simulink model "Lazurit_VD_3x_V1"  (R2018b)
settings: Solver=ode8  StartTime=0.0  StopTime=0.2  RelTol=1e-3
undefined symbols (not defined in the file): C_c, C_r, L_l, L_r, R, Us, Uzpt
libraries: powerlib x36, powerlib_meascontrol x10, peRmsMeasurement x4
settings Model: Creator=Anton  LastModifiedBy=VID Company
settings SFSimCC: SimUseLocalCustomCode=off
settings RTWCC: RTWUseLocalCustomCode=off
settings CodeAppCC: StateflowObjectComments=on
settings SimscapeCC: SimscapeNormalizeSystem=off

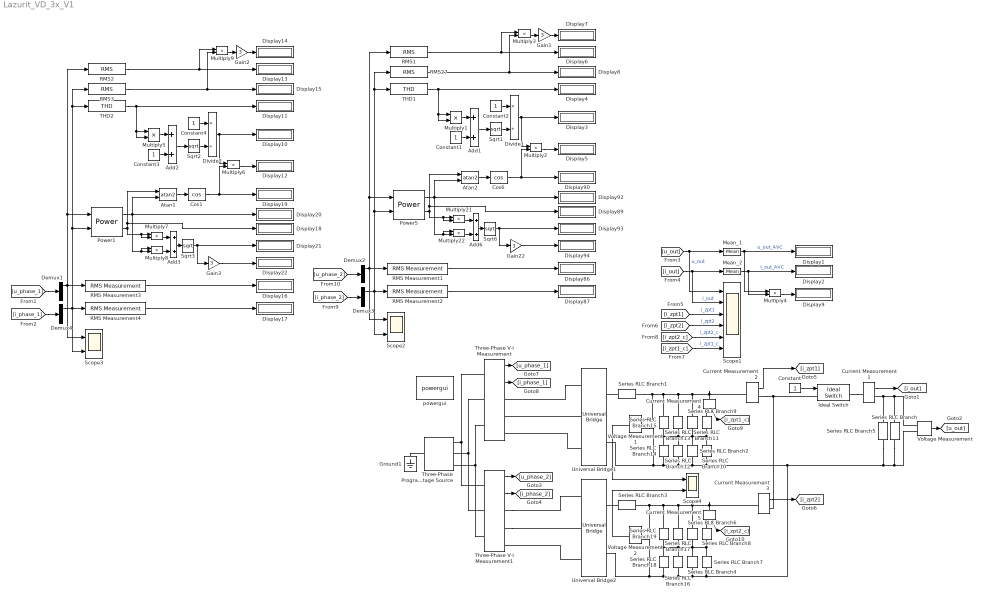
== system Lazurit_VD_3x_V1 ==
  Add{1..3,6} (4 alike) : Sum
  Atan1 : Trigonometry  Operator=atan2
  Atan2 : Trigonometry  Operator=atan2
  Constant{,1..4} (5 alike) : Constant
  Cos1 : Trigonometry  Operator=cos
  Cos6 : Trigonometry  Operator=cos
  Current Measurement{1..5} (5 alike) : powerlib/Measurements/Current Measurement  PhasorSimulation=off  OutputType=Complex  PSBequivalent=0
  Demux{1..4} (4 alike) : Demux  Outputs=3
  Display{1..22,86..87,89..90,92..94} (29 alike) : Display
  Divide1 : Product  Inputs=*/
  Divide2 : Product  Inputs=*/
  Gain{1..3,22} (4 alike) : Gain  Gain=3
  Ground1 : powerlib/Elements/Ground  LConnTagsString=a
  Ideal Switch : powerlib/Power Electronics/Ideal Switch  Ron=0.001  Lon=0  IC=0  Rs=1e5  Cs=inf  Measurements=off
  Mean_1 : powerlib_meascontrol/Measurements/Mean  Freq=300  Vinit=0  Ts=0
  Mean_2 : powerlib_meascontrol/Measurements/Mean  Freq=300  Vinit=0  Ts=0
  Multiply{1..9,21..22} (11 alike) : Product
  Power1 : powerlib_meascontrol/Measurements/Power  Freq=50  Vinit=[1, 0]  Iinit=[1, 0]  Ts=0
      settings: SourceProductName=Simscape Power Systems
  Power5 : powerlib_meascontrol/Measurements/Power  Freq=50  Vinit=[1, 0]  Iinit=[1, 0]  Ts=0
      settings: SourceProductName=Simscape Power Systems
  RMS Measurement{1..4} (4 alike) : peRmsMeasurement/RMS Measurement  LabelModeActiveChoice=Harmonic  F=50  SpecifyHarmonics=on  K=[1]  Ts=0
  RMS{1..3,27} (4 alike) : powerlib_meascontrol/Measurements/RMS  TrueRMS=on  Freq=50  RMSInit=0  Ts=0
  Scope1 : Scope  NumInputPorts=6
  Scope2 : Scope  NumInputPorts=2
  Scope3 : Scope  NumInputPorts=2
  Scope4 : Scope  NumInputPorts=2
  Series RLC Branch : powerlib/Elements/Series RLC Branch  LConnTagsString=__new0  RConnTagsString=__new0  BranchType=R  Resistance=R  Inductance=250e-6  SetiL0=off  InitialCurrent=0  Capacitance=1e-6  Setx0=off  InitialVoltage=0  Measurements=None
  Series RLC Branch1 : powerlib/Elements/Series RLC Branch  LConnTagsString=__new0  RConnTagsString=__new0  BranchType=RL  Resistance=L_r  Inductance=L_l  SetiL0=off  InitialCurrent=0  Capacitance=1e-6  Setx0=off  InitialVoltage=0  Measurements=None
  Series RLC Branch{2,4,6..19} (16 alike) : powerlib/Elements/Series RLC Branch  LConnTagsString=__new0  RConnTagsString=__new0  BranchType=RC  Resistance=C_r  Inductance=250e-6  SetiL0=off  InitialCurrent=0  Capacitance=C_c  Setx0=on  InitialVoltage=Uzpt/2  Measurements=None
  Series RLC Branch3 : powerlib/Elements/Series RLC Branch  LConnTagsString=__new0  RConnTagsString=__new0  BranchType=RL  Resistance=L_r  Inductance=L_l  SetiL0=off  InitialCurrent=0  Capacitance=1e-6  Setx0=off  InitialVoltage=0  Measurements=None
  Series RLC Branch5 : powerlib/Elements/Series RLC Branch  LConnTagsString=__new0  RConnTagsString=__new0  BranchType=R  Resistance=R  Inductance=250e-6  SetiL0=off  InitialCurrent=0  Capacitance=1e-6  Setx0=off  InitialVoltage=0  Measurements=None
  Sqrt{1..3,6} (4 alike) : Sqrt  SaturateOnIntegerOverflow=on
  THD1 : powerlib_meascontrol/Measurements/THD  Freq=50  Ts=0
  THD2 : powerlib_meascontrol/Measurements/THD  Freq=50  Ts=0
  Three-Phase Programmable Voltage Source : powerlib/Electrical Sources/Three-Phase Programmable Voltage Source  PositiveSequence=[Us 0 50]  VariationEntity=None  VariationType=Table of time-amplitude pairs  VariationTypeAlt=Step  VariationStep=0.5  VariationRate=10  VariationMagnitude=0.3  VariationFrequency=2  VariationTiming=[1 2]  VariationPhaseA=off  Amplitudes=[1 0.8 1.2 1.0]  TimeValues=[0 0.1 0.15 0.2]  HarmonicGeneration=off  HarmonicA=[3 0.2 -25 0]  HarmonicB=[2 0.15 35 2]  Timing="[0.05  3]"  BusType=swing  Pref=0  Qref=0  Qmin=-inf  Qmax=inf
  Three-Phase V-I Measurement : powerlib/Measurements/Three-Phase V-I Measurement  VoltageMeasurement=phase-to-ground  SetLabelV=off  LabelV=Vabc  Vpu=off  VpuLL=off  CurrentMeasurement=yes  SetLabelI=off  LabelI=Iabc  Ipu=off  Pbase=100e6  Vbase=500e3  OutputType=Complex  PhasorSimulation=off  PSBequivalent=0
  Three-Phase V-I Measurement1 : powerlib/Measurements/Three-Phase V-I Measurement  VoltageMeasurement=phase-to-ground  SetLabelV=off  LabelV=Vabc  Vpu=off  VpuLL=off  CurrentMeasurement=yes  SetLabelI=off  LabelI=Iabc  Ipu=off  Pbase=100e6  Vbase=500e3  OutputType=Complex  PhasorSimulation=off  PSBequivalent=0
  Universal Bridge1 : powerlib/Power Electronics/Universal Bridge  Arms=3  SnubberResistance=1e5  SnubberCapacitance=inf  Device=Diodes  Ron=5e-3  Lon=0  ForwardVoltages="[  0  0  ]"  ForwardVoltage=1.5  GTOparameters=[ 10e-6 , 20e-6 ]  IGBTparameters=[ 1e-6 , 2e-6 ]  Measurements=None  Measurements_2=None  converterType=Rectifier
  Universal Bridge2 : powerlib/Power Electronics/Universal Bridge  Arms=3  SnubberResistance=1e5  SnubberCapacitance=inf  Device=Diodes  Ron=5e-3  Lon=0  ForwardVoltages="[  0  0  ]"  ForwardVoltage=1.5  GTOparameters=[ 10e-6 , 20e-6 ]  IGBTparameters=[ 1e-6 , 2e-6 ]  Measurements=None  Measurements_2=None  converterType=Rectifier
  Voltage Measurement : powerlib/Measurements/Voltage Measurement  PhasorSimulation=off  OutputType=Complex  PSBequivalent=0
  Voltage Measurement1 : powerlib/Measurements/Voltage Measurement  PhasorSimulation=off  OutputType=Complex  PSBequivalent=0
  Voltage Measurement2 : powerlib/Measurements/Voltage Measurement  PhasorSimulation=off  OutputType=Complex  PSBequivalent=0
  powergui : powerlib/powergui  Priority=1  SimulationMode=Discrete  SampleTime=1e-6  frequency=60  Iterations=50  frequencyindice=0  Pbase=100e6  ErrMax=1e-4  UnitsV=kV  UnitsW=MW  buscounter=0  FunctionMessages=off  echomessages=off  EnableUseOfTLC=off  CurrentSourceSwitches=off  DisableSnubberDevices=off  DisableRonSwitches=off  DisableVfSwitches=off  DisplayEquations=off  SolverType=Tustin/Backward Euler (TBE)  Interpol=off  ExternalGateDelay=off  methode=off  Ts=100  x0status=blocks  SPID=off  SwTol=0  HookPort=off  RestoreLinks=warning  ResistiveCurrentMeasurement=off  Frange=[0:2:500]  Ylog=off  Xlog=on  ShowGrid=off  save=off  variable=ZData  structure=0  ZoomFFT=off  StartTime=0.0  cycles=1  DisplayStyle=1  fundamental=60  FreqAxis=off  MaxFrequency=1000  frequencyindicesteady=1  RmsSteady=1  display=off
  wires:
  Three-Phase V-I Measurement/2 -> [i_phase_1]
  Three-Phase V-I Measurement/1 -> [u_phase_1]
  [i_phase_2] -> Demux3/1
  Gain22/1 -> Display94/1
  Sqrt6/1 -> Display93/1, Gain22/1
  Demux2/1 -> Scope2/1, RMS Measurement1/1, RMS1/1, Power5/1
  Add6/1 -> Sqrt6/1
  Atan2/1 -> Cos6/1
  Power5/2 -> Atan2/1, Display89/1, Multiply21/2, Multiply21/1
  Demux3/1 -> Scope2/2, RMS Measurement2/1, THD1/1, RMS27/1, Power5/2
  Multiply21/1 -> Add6/1
  Cos6/1 -> Multiply2/2, Display90/1
  [u_phase_2] -> Demux2/1
  Multiply22/1 -> Add6/2
  RMS Measurement1/1 -> Display86/1
  RMS Measurement2/1 -> Display87/1
  Power5/1 -> Atan2/2, Multiply22/1, Multiply22/2, Display92/1
  Voltage Measurement/1 -> [u_out]
  [i_out] -> Mean_2/1, Scope1/2  "i_out"
  [u_out] -> Mean_1/1, Scope1/1  "u_out"
  Multiply1/1 -> Add1/1
  Constant2/1 -> Divide1/1
  Add1/1 -> Sqrt1/1
  Sqrt1/1 -> Divide1/2
  Divide1/1 -> Multiply2/1, Display3/1
  Constant1/1 -> Add1/2
  THD1/1 -> Multiply1/2, Multiply1/1, Display4/1
  RMS27/1 -> Multiply3/2, Display8/1
  Multiply2/1 -> Display5/1
  RMS1/1 -> Multiply3/1, Display6/1
  Gain1/1 -> Display7/1
  Multiply3/1 -> Gain1/1
  Mean_1/1 -> Display1/1, Multiply4/1  "u_out_AVC"
  Mean_2/1 -> Display2/1, Multiply4/2  "I_out_AVC"
  Multiply4/1 -> Display9/1
  Current Measurement1/1 -> [i_out]
  Three-Phase V-I Measurement1/1 -> [u_phase_2]
  Three-Phase V-I Measurement1/2 -> [i_phase_2]
  THD2/1 -> Multiply5/2, Multiply5/1, Display11/1
  Power1/2 -> Atan1/1, Display18/1, Multiply7/2, Multiply7/1
  Add2/1 -> Sqrt2/1
  RMS3/1 -> Multiply9/2, Display15/1
  Multiply6/1 -> Display12/1
  Multiply9/1 -> Gain2/1
  Demux1/1 -> Scope3/1, RMS Measurement3/1, RMS2/1, Power1/1
  Constant3/1 -> Add2/2
  RMS Measurement4/1 -> Display17/1
  RMS2/1 -> Multiply9/1, Display13/1
  Gain2/1 -> Display14/1
  Cos1/1 -> Multiply6/2, Display19/1
  Sqrt3/1 -> Display21/1, Gain3/1
  Multiply5/1 -> Add2/1
  Multiply7/1 -> Add3/1
  [u_phase_1] -> Demux1/1
  Multiply8/1 -> Add3/2
  Gain3/1 -> Display22/1
  Demux4/1 -> Scope3/2, RMS Measurement4/1, THD2/1, RMS3/1, Power1/2
  Constant4/1 -> Divide2/1
  Power1/1 -> Atan1/2, Multiply8/1, Multiply8/2, Display20/1
  Add3/1 -> Sqrt3/1
  RMS Measurement3/1 -> Display16/1
  Divide2/1 -> Multiply6/1, Display10/1
  [i_phase_1] -> Demux4/1
  Atan1/1 -> Cos1/1
  Sqrt2/1 -> Divide2/2
  Current Measurement2/1 -> [i_zpt1]
  Current Measurement3/1 -> [i_zpt2]
  [i_zpt1] -> Scope1/3  "i_zpt1"
  [i_zpt2] -> Scope1/4  "i_zpt2"
  Current Measurement5/1 -> [i_zpt2_c]
  Current Measurement4/1 -> [i_zpt1_c]
  [i_zpt2_c] -> Scope1/5  "i_zpt2_c"
  [i_zpt1_c] -> Scope1/6  "i_zpt1_c"
  Constant/1 -> Ideal Switch/1
  Voltage Measurement1/1 -> Scope4/1
  Voltage Measurement2/1 -> Scope4/2
  connections:
  Universal Bridge1/LConn1 -- Three-Phase V-I Measurement/RConn1
  Universal Bridge1/LConn3 -- Three-Phase V-I Measurement/RConn3
  Universal Bridge1/LConn2 -- Three-Phase V-I Measurement/RConn2
  Three-Phase Programmable Voltage Source/RConn1 -- Three-Phase V-I Measurement/LConn1 -- Three-Phase V-I Measurement1/LConn1
  Three-Phase Programmable Voltage Source/LConn1 -- Ground1/LConn1
  Three-Phase Programmable Voltage Source/RConn3 -- Three-Phase V-I Measurement/LConn3 -- Three-Phase V-I Measurement1/LConn3
  Three-Phase Programmable Voltage Source/RConn2 -- Three-Phase V-I Measurement/LConn2 -- Three-Phase V-I Measurement1/LConn2
  Series RLC Branch/RConn1 -- Voltage Measurement/LConn2 -- Series RLC Branch5/RConn1 -- Series RLC Branch16/RConn1 -- Series RLC Branch18/RConn1 -- Voltage Measurement2/LConn2 -- Universal Bridge2/RConn2 -- Series RLC Branch4/RConn1 -- Series RLC Branch7/RConn1 -- Series RLC Branch12/RConn1 -- Series RLC Branch14/RConn1 -- Voltage Measurement1/LConn2 -- Universal Bridge1/RConn2 -- Series RLC Branch2/RConn1 -- Series RLC Branch10/RConn1
  Voltage Measurement/LConn1 -- Series RLC Branch5/LConn1 -- Current Measurement1/RConn1 -- Series RLC Branch/LConn1
  Three-Phase V-I Measurement1/RConn1 -- Universal Bridge2/LConn1
  Three-Phase V-I Measurement1/RConn2 -- Universal Bridge2/LConn2
  Universal Bridge2/LConn3 -- Three-Phase V-I Measurement1/RConn3
  Current Measurement3/LConn1 -- Current Measurement5/LConn1 -- Series RLC Branch6/LConn1 -- Series RLC Branch17/LConn1 -- Series RLC Branch19/LConn1 -- Voltage Measurement2/LConn1 -- Series RLC Branch3/RConn1
  Series RLC Branch1/RConn1 -- Series RLC Branch15/LConn1 -- Series RLC Branch13/LConn1 -- Series RLC Branch9/LConn1 -- Current Measurement4/LConn1 -- Current Measurement2/LConn1 -- Voltage Measurement1/LConn1
  Current Measurement5/RConn1 -- Series RLC Branch8/LConn1
  Current Measurement2/RConn1 -- Ideal Switch/LConn1 -- Current Measurement3/RConn1
  Current Measurement4/RConn1 -- Series RLC Branch11/LConn1
  Series RLC Branch3/LConn1 -- Universal Bridge2/RConn1
  Series RLC Branch1/LConn1 -- Universal Bridge1/RConn1
  Ideal Switch/RConn1 -- Current Measurement1/LConn1
  Series RLC Branch11/RConn1 -- Series RLC Branch10/LConn1 -- Series RLC Branch12/LConn1 -- Series RLC Branch13/RConn1 -- Series RLC Branch14/LConn1 -- Series RLC Branch15/RConn1 -- Series RLC Branch2/LConn1 -- Series RLC Branch9/RConn1
  Series RLC Branch6/RConn1 -- Series RLC Branch16/LConn1 -- Series RLC Branch17/RConn1 -- Series RLC Branch18/LConn1 -- Series RLC Branch19/RConn1 -- Series RLC Branch8/RConn1 -- Series RLC Branch7/LConn1 -- Series RLC Branch4/LConn1
